simulink model "sym5"  (R2022b)
settings: Solver=VariableStepAuto  StartTime=0.0  StopTime=50  RelTol=1e-3
values from neighbouring files (symbols this model uses):
  Hf = tf(Kp, [T1*T2 T1+T2 1], 'IoDelay', Tm)    [Lab5.m]
  Hkc1 = Q/(1-P)    [Lab5.m]
  Hkc2 = Hkc1    [Lab5.m]
  Hkc3 = minreal(Hkc2*num/sum(num.num{1,1})*den/sum(den.num{1,1}))    [Lab5.m]
  k = Tm    (= 3)    [Lab5.m]
settings Model: Creator=Pacuraru Fabian  LastModifiedBy=Pacuraru Fabian

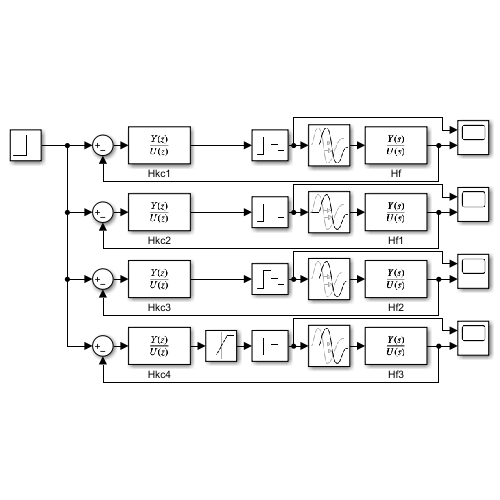
[thumbnail: Simulink's stored preview of the top-level diagram]
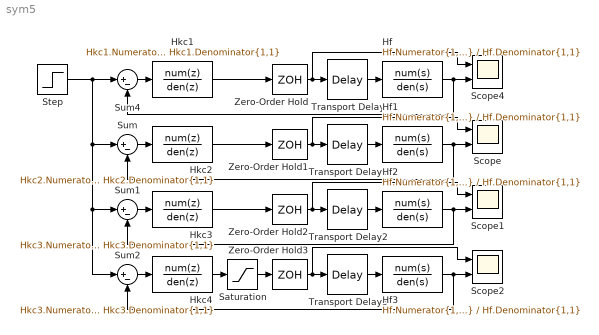
== system sym5 ==
  Hf{,1..3} (4 alike) : TransferFcn  Numerator=Hf.Numerator{1,1}  Denominator=Hf.Denominator{1,1}
  Hkc1 : DiscreteTransferFcn  Numerator=Hkc1.Numerator{1,1}  Denominator=Hkc1.Denominator{1,1}
  Hkc2 : DiscreteTransferFcn  Numerator=Hkc2.Numerator{1,1}  Denominator=Hkc2.Denominator{1,1}
  Hkc3 : DiscreteTransferFcn  Numerator=Hkc3.Numerator{1,1}  Denominator=Hkc3.Denominator{1,1}
  Hkc4 : DiscreteTransferFcn  Numerator=Hkc3.Numerator{1,1}  Denominator=Hkc3.Denominator{1,1}
  Saturation : Saturate  UpperLimit=5  LowerLimit=0
  Scope{,1..2,4} (4 alike) : Scope  NumInputPorts=2
  Step : Step  Time=0  SampleTime=0
  Sum{,1..2,4} (4 alike) : Sum  Inputs=|+-
  Transport Delay{,1..3} (4 alike) : TransportDelay  DelayTime=k
  Zero-Order Hold{,1..3} (4 alike) : ZeroOrderHold  SampleTime=-1
  wires:
  Hkc1/1 -> Zero-Order Hold/1
  Transport Delay/1 -> Hf/1
  Zero-Order Hold/1 -> Transport Delay/1, Scope4/1
  Hf/1 -> Sum4/2, Scope4/2
  Sum4/1 -> Hkc1/1
  Hkc2/1 -> Zero-Order Hold1/1
  Transport Delay1/1 -> Hf1/1
  Zero-Order Hold1/1 -> Transport Delay1/1, Scope/1
  Hf1/1 -> Sum/2, Scope/2
  Sum/1 -> Hkc2/1
  Step/1 -> Sum4/1, Sum/1, Sum1/1, Sum2/1
  Hkc3/1 -> Zero-Order Hold2/1
  Transport Delay2/1 -> Hf2/1
  Zero-Order Hold2/1 -> Transport Delay2/1, Scope1/1
  Hf2/1 -> Sum1/2, Scope1/2
  Sum1/1 -> Hkc3/1
  Transport Delay3/1 -> Hf3/1
  Zero-Order Hold3/1 -> Transport Delay3/1, Scope2/1
  Hf3/1 -> Sum2/2, Scope2/2
  Sum2/1 -> Hkc4/1
  Hkc4/1 -> Saturation/1
  Saturation/1 -> Zero-Order Hold3/1
